simulink model "quadcopter_rotation_subsystem"  (R2023b)
settings: Solver=ode3  StartTime=0  StopTime=inf  FixedStep=0.005  RelTol=1e-3  EnableMultiTasking=on
values from neighbouring files (symbols this model uses):
  alpha_vect = A\B    [poly3traj.m]
  g = 9.81    [MRB.m]
  Ic = [Ixx,0,0;0,Iyy,0;0,0,Izz]    [MRB.m]
  m = 4    [MRB.m]
  Mrb = [m*eye(3),zeros(3);zeros(3),Ic]    [MRB.m]
libraries: aerolibutil x11, simulink_extras x10, slpidlib x6, sharedtransform x3, sharedutil x2, vrlib x2
(part 1 of 2)
settings Model: Creator=The MathWorks, Inc.  LastModifiedBy=branko
settings SolverCC: AlgebraicLoopSolver=TrustRegion
settings DataIOCC: LimitDataPoints=on  SaveFormat=Array  SaveOutput=off  SignalLogging=off  DSMLogging=off  SaveTime=off  ReturnWorkspaceOutputs=off
settings OptimizationCC: BlockReduction=off  BufferReuse=off  LifeSpan=inf
settings DebuggingCC: AlgebraicLoopMsg=none  ParameterPrecisionLossMsg=none  AllowSymbolicDim=off  PregeneratedLibrarySubsystemCodeDiagnostic=none  SFUnexpectedBacktrackingDiag=warning  SFNoUnconditionalDefaultTransitionDiag=warning  SFExecutionAtInitializationDiag=none  ArithmeticOperatorsInVariantConditions=warning
settings HardwareCC: ProdBitPerPointer=32  ProdBitPerSizeT=32  ProdBitPerPtrDiffT=32  ProdLargestAtomicFloat=None  ProdIntDivRoundTo=Undefined  ProdEndianess=Unspecified  ProdWordSize=32  ProdHWDeviceType=32-bit Generic
settings ModelReferenceCC: EnableRefExpFcnMdlSchedulingChecks=on  PropagateSignalLabelsOutOfModel=off
settings SFSimCC: SimUseLocalCustomCode=off  CustomCodeUndefinedFunction=UseInterfaceOnly
settings RTWCC: RTWUseLocalCustomCode=off  DLArmComputeVersion=19.05
settings CodeAppCC: StateflowObjectComments=on
settings GRTTargetCC: TargetLangStandard=C89/C90 (ANSI)
settings ConfigComp: CovMetricSettings=dw  CovSaveCumulativeToWorkspaceVar=on  CovSaveSingleToWorkspaceVar=on  CovExternalEMLEnable=off  CovSFcnEnable=off

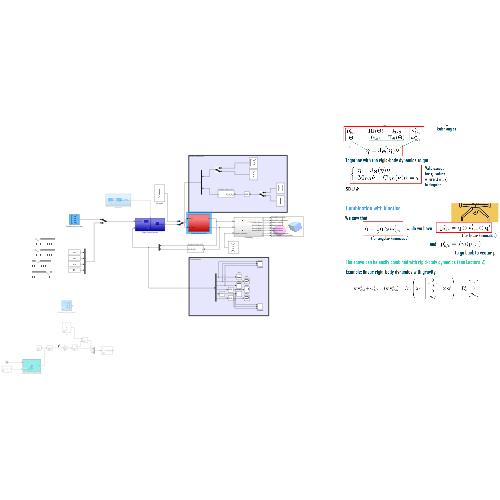
[thumbnail: Simulink's stored preview of the top-level diagram]
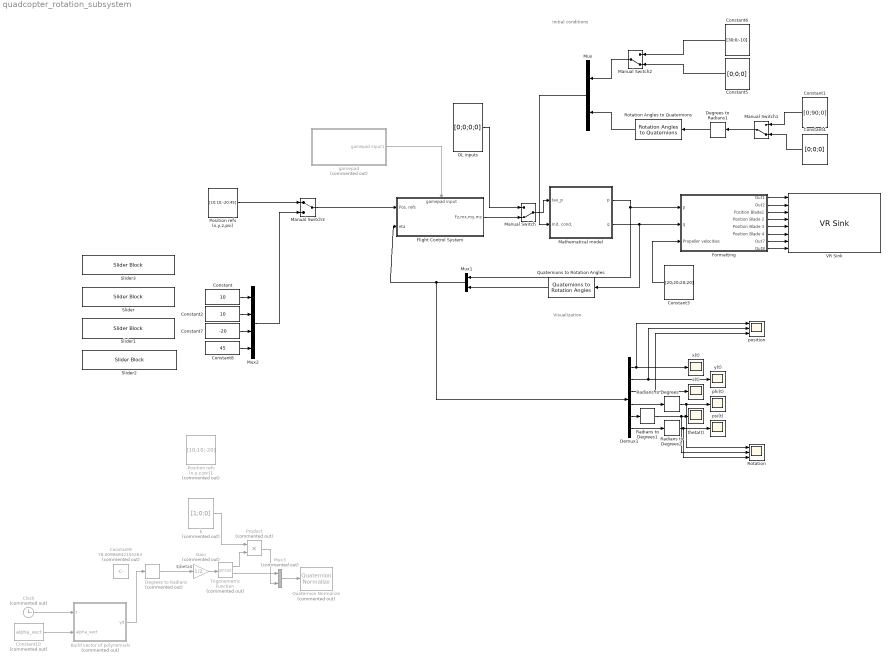
== system quadcopter_rotation_subsystem ==
  note: Visualization
  note: Initial conditions
  note: $\beta$
  Build vector of polynomials : MATLAB Function  Commented=on  TreatAsAtomicUnit=on
  Clock : Clock  Commented=on
  Constant : Constant  Value=10
  Constant1 : Constant  Value=[0;90;0]  VectorParams1D=off
  Constant10 : Constant  Commented=on  Value=alpha_vect  VectorParams1D=off
  Constant2 : Constant  Value=10
  Constant3 : Constant  Value=[20;20;20;20]  VectorParams1D=off
  Constant4 : Constant  Value=[0;0;0]  VectorParams1D=off
  Constant5 : Constant  Value=[0;0;0]  VectorParams1D=off
  Constant6 : Constant  Value=[30;0;-10]  VectorParams1D=off
  Constant7 : Constant  Value=-20
  Constant8 : Constant  Value=45
  Constant9 : Constant  Commented=on  Value=78.00986842105263
  Degrees to Radians : simulink_extras/Transformations/Degrees to Radians  Commented=on
  Degrees to Radians1 : simulink_extras/Transformations/Degrees to Radians
  Demux1 : Demux  Outputs=6
  Flight Control System : Subsystem
      settings: PortSchema="{\"entries\":[{\"content\":{\"sides\":[{\"content\":{\"connectorIds\":[\"In1\",\"In2\"]},\"type\":\"ConnectorPlacement.EquallySpacedRectSide\",\"uuid\":\"8ffec179-99fb-4b4c-a09d-a73fa0154dea\"},{\"content\":{\"connectorIds\":[\"Out1\"],\"side\":\"RIGHT\"},\"type\":\"ConnectorPlacement.EquallySpacedRectSide\",\"uuid\":\"b9ff487d-1da1-449a-81c9-f1838b0d3727\"},{\"content\":{\"connectorIds\":[\"In3\"],\"side\":\"TOP\"},\"type\":\"ConnectorPlacement.EquallySpacedRectSide\",\"uuid\":\"1948ac9a-8b1f-4a62-833b-18e2b106d39d\"}]},\"type\":\"ConnectorPlacement.EquallySpacedConnector\",\"uuid\":\"fea635f7-9753-4696-bad7-e2485c1b5acc\"}],\"packageUris\":[\"http://schema.mathworks.com/mf0/Connector/R2020b\"],\"version\":\"1.0\"}"
  Formatting : Subsystem
  Gain : Gain  Commented=on  Gain=1/2
  Manual Switch : ManualSwitch  CurrentSetting=0
  Manual Switch1 : ManualSwitch  CurrentSetting=0
  Manual Switch2 : ManualSwitch  CurrentSetting=0
  Manual Switch3 : ManualSwitch
  Mathematical model : Subsystem
  Mux : Mux  Inputs=2
  Mux1 : Mux  Inputs=2
  Mux2 : Mux
  Mux3 : Mux  Commented=on  Inputs=2
  OL inputs : Constant  Value=[0;0;0;0]  VectorParams1D=off
  Position refs (x,y,z,psi) : Constant  Value=[10;10;-20;45]  VectorParams1D=off
  Position refs (x,y,z,psi)1 : Constant  Commented=on  Value=[10;10;-20]  VectorParams1D=off
  Product : Product  Commented=on
  Quaternion Normalize : sharedutil/Quaternion Normalize  Commented=on  aMode=aMode
  Quaternions to Rotation Angles : sharedtransform/Quaternions to Rotation Angles  rotationOrder=XYZ  aMode=aMode
  Radians to Degrees : simulink_extras/Transformations/Radians to Degrees
  Radians to Degrees1 : simulink_extras/Transformations/Radians to Degrees
  Radians to Degrees2 : simulink_extras/Transformations/Radians to Degrees
  Rotation : Scope  NumInputPorts=3
  Rotation Angles to Quaternions : sharedtransform/Rotation Angles to Quaternions  rotationOrder=XYZ  aMode=aMode
  Slider : SliderBlock
  Slider1 : SliderBlock  ScaleMin=-50  ScaleMax=50
  Slider2 : SliderBlock  ScaleMin=-65  ScaleMax=65
  Slider3 : SliderBlock
  Trigonometric Function : Trigonometry  Commented=on  Operator=sincos
  VR Sink : vrlib/VR Sink  InstantiateOnLoad=on  SampleTime=12*0.005  ViewEnable=on  RemoteChange=off  RemoteView=off  FieldsWritten=QuadBody.rotation.4.1.1.double#QuadBody.translation.3.1.1.double#Blade1.rotation.4.1.1.double#Blade3.rotation.4.1.1.double#Blade2.rotation.4.1.1.double#Blade4.rotation.4.1.1.double#IsoNoRotation.position.3.1.1.double#OnQuadNoRotation.position.3.1.1.double  WorldFileName=Quadcopter_VR.wrl  AutoView=on  VideoDimensions=[]  AllowVariableSize=off
  gamepad : Subsystem  Commented=on
  k : Constant  Commented=on  Value=[1;0;0]  VectorParams1D=off
  phi(t) : Scope
  position : Scope  NumInputPorts=3
  psi(t) : Scope
  theta(t) : Scope
  x(t) : Scope
  y(t) : Scope
  z(t) : Scope
  wires:
  Formatting/5(Position Blade 3) -> VR Sink/5
  Formatting/7(Out7) -> VR Sink/7
  Formatting/6(Position Blade 4) -> VR Sink/6
  Formatting/3(Position Blade1) -> VR Sink/3
  Formatting/1(Out1) -> VR Sink/1
  Formatting/4(Position Blade 2) -> VR Sink/4
  Formatting/2(Out2) -> VR Sink/2
  Formatting/8(Out8) -> VR Sink/8
  Constant3/1 -> Formatting/3(Propeller velocities)
  OL inputs/1 -> Manual Switch/1
  Flight Control System/1(Fz,mx,my,mz) -> Manual Switch/2
  Manual Switch2/1 -> Mux/1
  Rotation Angles to Quaternions/1 -> Mux/2
  gamepad/1(gamepad input1) -> Flight Control System/3(gamepad input)
  Mathematical model/1(p) -> Mux1/1, Formatting/1(p)
  Mathematical model/2(q) -> Formatting/2(q), Quaternions to Rotation Angles/1
  Mux/1 -> Mathematical model/2(Init. cond.)
  Constant6/1 -> Manual Switch2/1
  Constant5/1 -> Manual Switch2/2
  Manual Switch1/1 -> Degrees to Radians1/1
  Degrees to Radians1/1 -> Rotation Angles to Quaternions/1
  Constant1/1 -> Manual Switch1/1
  Constant4/1 -> Manual Switch1/2
  Quaternions to Rotation Angles/1 -> Mux1/2
  Mux1/1 -> Demux1/1, Flight Control System/2(eta)
  Demux1/5 -> Radians to Degrees1/1
  Demux1/6 -> Radians to Degrees2/1
  Demux1/2 -> position/2, y(t)/1
  Demux1/3 -> z(t)/1, position/3
  Radians to Degrees/1 -> Rotation/1, phi(t)/1
  Demux1/1 -> position/1, x(t)/1
  Radians to Degrees1/1 -> Rotation/2, theta(t)/1
  Radians to Degrees2/1 -> Rotation/3, psi(t)/1
  Demux1/4 -> Radians to Degrees/1
  Constant8/1 -> Mux2/4
  Constant7/1 -> Mux2/3
  Constant/1 -> Mux2/1
  Constant2/1 -> Mux2/2
  Mux2/1 -> Manual Switch3/2
  Manual Switch3/1 -> Flight Control System/1(Pos. refs)
  Trigonometric Function/1 -> Product/2
  Build vector of polynomials/1(yd) -> Degrees to Radians/1
  Mux3/1 -> Quaternion Normalize/1
  Trigonometric Function/2 -> Mux3/1
  Constant10/1 -> Build vector of polynomials/2(alpha_vect)
  Product/1 -> Mux3/2
  Clock/1 -> Build vector of polynomials/1(t)
  Gain/1 -> Trigonometric Function/1
  k/1 -> Product/1
  Degrees to Radians/1 -> Gain/1
  Position refs (x,y,z,psi)/1 -> Manual Switch3/1
  Manual Switch/1 -> Mathematical model/1(tau_p)

== system quadcopter_rotation_subsystem/Flight Control System ==
  Pos. refs : Inport
  eta : Inport  Port=2
  gamepad input : Inport  Port=3
  Inner-loop PID controllers : Subsystem
  Manual Switch : ManualSwitch  CurrentSetting=0
  Outer loop position control : Subsystem
  m_y(t) : Scope
  Fz,mx,my,mz : Outport
  wires:
  Inner-loop PID controllers/1(Fz,mx,my,mz) -> Fz,mx,my,mz/1
  Manual Switch/1 -> Inner-loop PID controllers/1(desired z,phi,theta,psi)
  eta/1 -> Outer loop position control/2(eta), Inner-loop PID controllers/2(eta)
  Pos. refs/1 -> Outer loop position control/1(Pos. refs)
  Outer loop position control/1(desired z,phi,theta,psi) -> Manual Switch/2
  gamepad input/1 -> Manual Switch/1

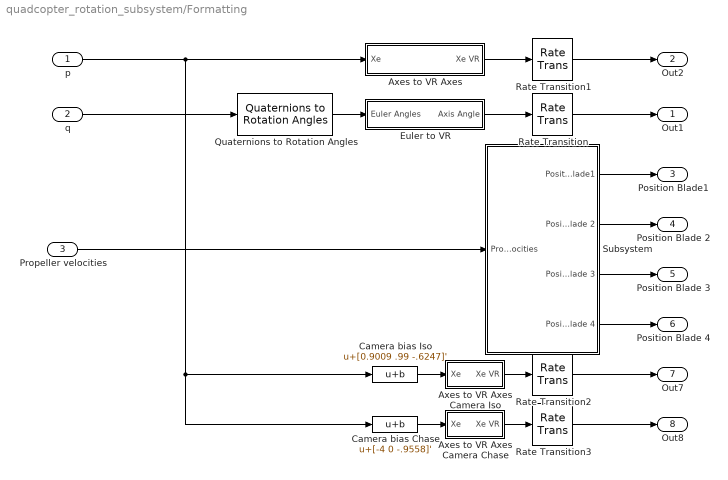
== system quadcopter_rotation_subsystem/Formatting ==
  p : Inport
  q : Inport  Port=2
  Propeller velocities : Inport  Port=3
  Axes to VR Axes : Subsystem
  Axes to VR Axes Camera Chase : Subsystem
  Axes to VR Axes Camera Iso : Subsystem
  Camera bias Chase : Bias  Bias=[-4 0 -.9558]'  SaturateOnIntegerOverflow=off
  Camera bias Iso : Bias  Bias=[0.9009 .99 -.6247]'  SaturateOnIntegerOverflow=off
  Euler to VR : Subsystem
  Quaternions to Rotation Angles : sharedtransform/Quaternions to Rotation Angles  rotationOrder=XYZ  aMode=aMode
  Rate Transition{,1..3} (4 alike) : RateTransition
  Subsystem : Subsystem
  Out1 : Outport
  Out2 : Outport  Port=2
  Position Blade1 : Outport  Port=3
  Position Blade 2 : Outport  Port=4
  Position Blade 3 : Outport  Port=5
  Position Blade 4 : Outport  Port=6
  Out7 : Outport  Port=7
  Out8 : Outport  Port=8
  wires:
  Rate Transition2/1 -> Out7/1
  Propeller velocities/1 -> Subsystem/1(Propeller velocities)
  Subsystem/3(Position Blade 3) -> Position Blade 3/1
  Subsystem/1(Position Blade1) -> Position Blade1/1
  Camera bias Chase/1 -> Axes to VR Axes Camera Chase/1(Xe)
  Axes to VR Axes Camera Chase/1(Xe VR) -> Rate Transition3/1
  Subsystem/2(Position Blade 2) -> Position Blade 2/1
  Axes to VR Axes Camera Iso/1(Xe VR) -> Rate Transition2/1
  Euler to VR/1(Axis Angle) -> Rate Transition/1
  Axes to VR Axes/1(Xe VR) -> Rate Transition1/1
  Rate Transition1/1 -> Out2/1
  Camera bias Iso/1 -> Axes to VR Axes Camera Iso/1(Xe)
  Rate Transition3/1 -> Out8/1
  Rate Transition/1 -> Out1/1
  Subsystem/4(Position Blade 4) -> Position Blade 4/1
  Quaternions to Rotation Angles/1 -> Euler to VR/1(Euler Angles)
  q/1 -> Quaternions to Rotation Angles/1
  p/1 -> Camera bias Chase/1, Camera bias Iso/1, Axes to VR Axes/1(Xe)

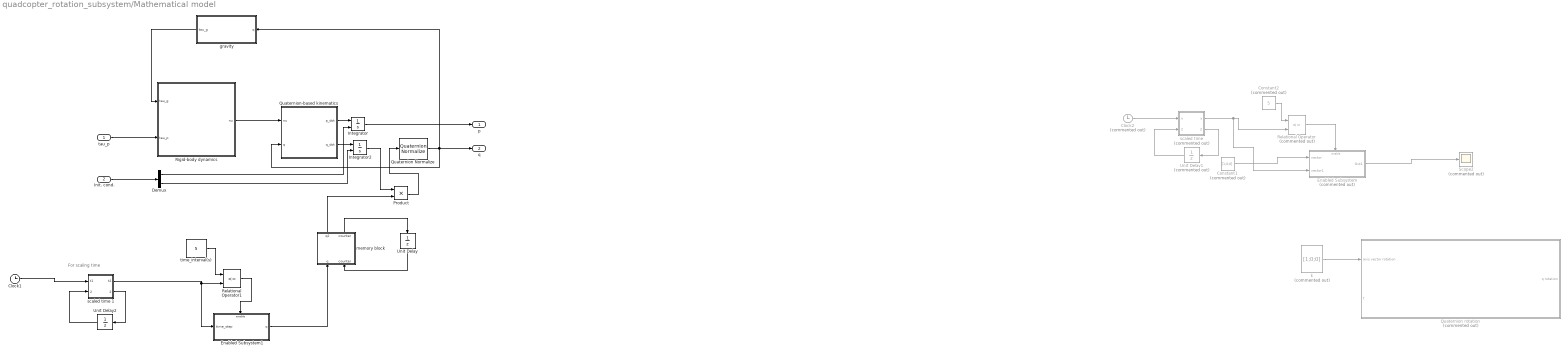
== system quadcopter_rotation_subsystem/Mathematical model ==
  note: For scaling time
  tau_p : Inport
  Init. cond. : Inport  Port=2
  " memory block" : MATLAB Function  TreatAsAtomicUnit=on
  Clock1 : Clock
  Clock2 : Clock  Commented=on
  Constant1 : Constant  Commented=on  Value=[1;0;0]
  Constant2 : Constant  Commented=on  Value=5
  Demux : Demux  Outputs=[3,4]
  Enabled Subsystem : Subsystem  Commented=on  TreatAsAtomicUnit=on
  Enabled Subsystem1 : Subsystem  TreatAsAtomicUnit=on
  Integrator : Integrator  InitialConditionSource=external  InitialCondition=[0;0;-10]
  Integrator2 : Integrator  InitialConditionSource=external  InitialCondition=[0;0;-10;0;pi/2;0]
  Product : Product
  Quaternion Normalize : sharedutil/Quaternion Normalize  aMode=aMode
  "Quaternion rotation " : Subsystem  Commented=on
  Quaternion-based kinematics : Subsystem
  Relational Operator : RelationalOperator  Commented=on  Operator=<=  OutDataTypeStr=boolean  RndMeth=Simplest  InputSameDT=off
  Relational Operator1 : RelationalOperator  Operator=<=  OutDataTypeStr=boolean  RndMeth=Simplest  InputSameDT=off
  Rigid-body dynamics : Subsystem
  Scope2 : Scope  Commented=on
  Unit Delay : UnitDelay  SampleTime=-1  HasFrameUpgradeWarning=on
  Unit Delay1 : UnitDelay  Commented=on  InitialCondition=[0 25]  SampleTime=0.01  HasFrameUpgradeWarning=on
  Unit Delay2 : UnitDelay  InitialCondition=[0 5]  SampleTime=-1  HasFrameUpgradeWarning=on
  gravity : Subsystem
  k : Constant  Commented=on  Value=[1;0;0]  VectorParams1D=off
  "scaled time " : MATLAB Function  Commented=on  TreatAsAtomicUnit=on
  scaled time 1 : MATLAB Function  TreatAsAtomicUnit=on
  time_interval(s) : Constant  Value=5
  p : Outport
  q : Outport  Port=2
  wires:
  Integrator/1 -> p/1
  Quaternion-based kinematics/1(p_dot) -> Integrator/1
  Quaternion Normalize/1 -> gravity/1(q), q/1, Quaternion-based kinematics/2(q)
  tau_p/1 -> Rigid-body dynamics/2(tau_p)
  Rigid-body dynamics/1(nu) -> Quaternion-based kinematics/1(nu)
  gravity/1(tau_g) -> Rigid-body dynamics/1(tau_g)
  Init. cond./1 -> Demux/1
  Demux/2 -> Integrator2/2
  Demux/1 -> Integrator/2
  Quaternion-based kinematics/2(q_dot) -> Integrator2/1
  Constant2/1 -> Relational Operator/1
  Enabled Subsystem/1(Out1) -> Scope2/1
  Unit Delay1/1 -> "scaled time "/2("counter_timer ")
  Relational Operator/1 -> Enabled Subsystem/Enable
  "scaled time "/1(y) -> Enabled Subsystem/2(vector1), Relational Operator/2
  "scaled time "/2(counter_timer) -> Unit Delay1/1
  Constant1/1 -> Enabled Subsystem/1(vector)
  Clock2/1 -> "scaled time "/1(u)
  k/1 -> "Quaternion rotation "/1(axis vector rotation)
  Clock1/1 -> scaled time 1/1(t1)
  time_interval(s)/1 -> Relational Operator1/1
  Relational Operator1/1 -> Enabled Subsystem1/Enable
  scaled time 1/1(t2) -> Enabled Subsystem1/1(time_step), Relational Operator1/2
  scaled time 1/2(counter_timer) -> Unit Delay2/1
  Unit Delay2/1 -> scaled time 1/2("counter_timer ")
  Enabled Subsystem1/1(q) -> " memory block"/1(q)
  Product/1 -> Quaternion Normalize/1
  Integrator2/1 -> Product/1
  " memory block"/1(q2) -> Product/2
  Unit Delay/1 -> " memory block"/2("counter ")
  " memory block"/2(counter) -> Unit Delay/1

== system quadcopter_rotation_subsystem/gamepad ==
  Formatting1 : Subsystem
  Gamepad1 : vrlib/Joystick Input  joyid=1  adjustports=on  forcefeed=off
  gamepad input1 : Outport
  wires:
  ? -> Formatting1/3(Point of View)
  Gamepad1/1 -> Formatting1/1(Axes)
  Formatting1/1(gamepad input) -> gamepad input1/1
  Gamepad1/2 -> Formatting1/2(Buttons)

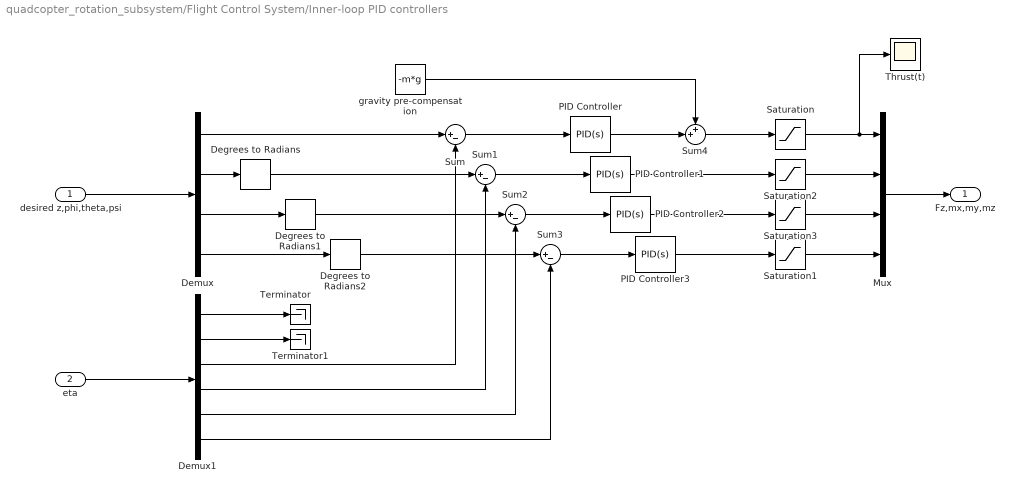
== system quadcopter_rotation_subsystem/Flight Control System/Inner-loop PID controllers ==
  desired z,phi,theta,psi : Inport
  eta : Inport  Port=2
  Degrees to Radians : simulink_extras/Transformations/Degrees to Radians
  Degrees to Radians1 : simulink_extras/Transformations/Degrees to Radians
  Degrees to Radians2 : simulink_extras/Transformations/Degrees to Radians
  Demux : Demux
  Demux1 : Demux  Outputs=6
  Mux : Mux
  PID Controller : slpidlib/PID Controller  Controller=PID  Form=Parallel  TimeDomain=Continuous-time  UseExternalTs=off  SampleTime=-1  IntegratorMethod=Forward Euler  FilterMethod=Forward Euler  ControllerParametersSource=internal  P=0.742717053084559  I=0.0347701341647605  UseKiTs=off  D=3.89568392639278  N=5.45397025421619  UseFilter=on  TunerSelectOption=Transfer Function Based (PID Tuner App)  InitialConditionSource=internal  InitialConditionForIntegrator=0  InitialConditionForFilter=0  DifferentiatorICPrevScaledInput=0  ExternalReset=none  TrackingMode=off  Kt=1  LimitOutput=off  SatLimitsSource=internal  UpperSaturationLimit=100  LowerSaturationLimit=-100  LinearizeAsGain=on  AntiWindupMode=none  Kb=1  LimitIntegrator=off  UpperIntegratorSaturationLimit=inf  LowerIntegratorSaturationLimit=-inf  POutMin=[]  POutMax=[]  IOutMin=[]  IOutMax=[]  DOutMin=[]  DOutMax=[]  NOutMin=[]  NOutMax=[]  SumOutMin=[]  SumOutMax=[]  SaturationOutMin=[]  SaturationOutMax=[]  PParamMin=[]  PParamMax=[]  IParamMin=[]  IParamMax=[]  DParamMin=[]  DParamMax=[]  NParamMin=[]  NParamMax=[]  KbParamMin=[]  KbParamMax=[]  KtParamMin=[]  KtParamMax=[]  KbOutMin=[]  KbOutMax=[]  KtOutMin=[]  KtOutMax=[]  IntegratorOutMin=[]  IntegratorOutMax=[]  FilterOutMin=[]  FilterOutMax=[]  SumI1OutMin=[]  SumI1OutMax=[]  SumI2OutMin=[]  SumI2OutMax=[]  SumI3OutMin=[]  SumI3OutMax=[]  SumI4OutMin=[]  SumI4OutMax=[]  SumDOutMin=[]  SumDOutMax=[]  DifferentiatorOutMin=[]  DifferentiatorOutMax=[]  FilterDiffOutCoefMin=[]  FilterDiffOutCoefMax=[]  ReciprocalOutMin=[]  ReciprocalOutMax=[]  SumDenOutMin=[]  SumDenOutMax=[]  SumNumOutMin=[]  SumNumOutMax=[]  DivideOutMin=[]  DivideOutMax=[]  UdiffTsProdOutMin=[]  UdiffTsProdOutMax=[]  NTsProdOutMin=[]  NTsProdOutMax=[]  UintegralTsProdOutMin=[]  UintegralTsProdOutMax=[]  UngainTsProdOutMin=[]  UngainTsProdOutMax=[]  ClampingZeroOutDataTypeStr=Inherit: Inherit via back propagation  ClampingZeroOutMin=[]  ClampingZeroOutMax=[]  FilterDenConstantOutDataTypeStr=Inherit: Inherit via back propagation  FilterDenConstantOutMin=[]  FilterDenConstantOutMax=[]  PCopyOutDataTypeStr=Inherit: Inherit via back propagation  PCopyOutMin=[]  PCopyOutMax=[]  NCopyOutDataTypeStr=Inherit: Inherit via back propagation  NCopyOutMin=[]  NCopyOutMax=[]  IntegratorContinuousStateAttributes=''  IntegratorStateMustResolveToSignalObject=off  IntegratorRTWStateStorageClass=Auto  FilterContinuousStateAttributes=''  FilterStateMustResolveToSignalObject=off  FilterRTWStateStorageClass=Auto  ParallelPVariant=InternalParameters  IdealPVariant=Disabled  IVariant=InternalParameters  DVariant=InternalParameters  IntegratorVariant=Continuous  SatVariant=Disabled  AWVariant=Passthrough  PCopyVariant=Disabled  TRVariant=Disabled  FdbkBlocksVariant=Forward  IdealPFdbkVariant=Disabled  SatFdbkVariant=Disabled  DerivativeFilterVariant=ContFilter  NVariant=InternalParameters  NCopyVariant=Disabled  FilterICVariant=InternalICsFilter  IntegratorICVariant=InternalICs  ExternalResetVariant=Disabled  TRSumVariant=Passthrough  SumFdbkVariant=Disabled  SumVariant=Sum_PID  TsampFilterVariant=InternalTs  TsampNgainVariant=Passthrough  TsampIntegralVariant=Disabled_SignalSpec  ExternalSaturationOutDataTypeStr=Inherit: Same as second input
  PID Controller1 : slpidlib/PID Controller  Controller=PID  Form=Parallel  TimeDomain=Continuous-time  UseExternalTs=off  SampleTime=-1  IntegratorMethod=Forward Euler  FilterMethod=Forward Euler  ControllerParametersSource=internal  P=38.1552916307711  I=12.5176201301645  UseKiTs=off  D=17.8958394627173  N=96.5468649773944  UseFilter=on  TunerSelectOption=Transfer Function Based (PID Tuner App)  InitialConditionSource=internal  InitialConditionForIntegrator=0  InitialConditionForFilter=0  DifferentiatorICPrevScaledInput=0  ExternalReset=none  TrackingMode=off  Kt=1  LimitOutput=off  SatLimitsSource=internal  UpperSaturationLimit=inf  LowerSaturationLimit=-inf  LinearizeAsGain=on  AntiWindupMode=none  Kb=1  LimitIntegrator=off  UpperIntegratorSaturationLimit=inf  LowerIntegratorSaturationLimit=-inf  POutMin=[]  POutMax=[]  IOutMin=[]  IOutMax=[]  DOutMin=[]  DOutMax=[]  NOutMin=[]  NOutMax=[]  SumOutMin=[]  SumOutMax=[]  SaturationOutMin=[]  SaturationOutMax=[]  PParamMin=[]  PParamMax=[]  IParamMin=[]  IParamMax=[]  DParamMin=[]  DParamMax=[]  NParamMin=[]  NParamMax=[]  KbParamMin=[]  KbParamMax=[]  KtParamMin=[]  KtParamMax=[]  KbOutMin=[]  KbOutMax=[]  KtOutMin=[]  KtOutMax=[]  IntegratorOutMin=[]  IntegratorOutMax=[]  FilterOutMin=[]  FilterOutMax=[]  SumI1OutMin=[]  SumI1OutMax=[]  SumI2OutMin=[]  SumI2OutMax=[]  SumI3OutMin=[]  SumI3OutMax=[]  SumI4OutMin=[]  SumI4OutMax=[]  SumDOutMin=[]  SumDOutMax=[]  DifferentiatorOutMin=[]  DifferentiatorOutMax=[]  FilterDiffOutCoefMin=[]  FilterDiffOutCoefMax=[]  ReciprocalOutMin=[]  ReciprocalOutMax=[]  SumDenOutMin=[]  SumDenOutMax=[]  SumNumOutMin=[]  SumNumOutMax=[]  DivideOutMin=[]  DivideOutMax=[]  UdiffTsProdOutMin=[]  UdiffTsProdOutMax=[]  NTsProdOutMin=[]  NTsProdOutMax=[]  UintegralTsProdOutMin=[]  UintegralTsProdOutMax=[]  UngainTsProdOutMin=[]  UngainTsProdOutMax=[]  ClampingZeroOutDataTypeStr=Inherit: Inherit via back propagation  ClampingZeroOutMin=[]  ClampingZeroOutMax=[]  FilterDenConstantOutDataTypeStr=Inherit: Inherit via back propagation  FilterDenConstantOutMin=[]  FilterDenConstantOutMax=[]  PCopyOutDataTypeStr=Inherit: Inherit via back propagation  PCopyOutMin=[]  PCopyOutMax=[]  NCopyOutDataTypeStr=Inherit: Inherit via back propagation  NCopyOutMin=[]  NCopyOutMax=[]  IntegratorContinuousStateAttributes=''  IntegratorStateMustResolveToSignalObject=off  IntegratorRTWStateStorageClass=Auto  FilterContinuousStateAttributes=''  FilterStateMustResolveToSignalObject=off  FilterRTWStateStorageClass=Auto  ParallelPVariant=InternalParameters  IdealPVariant=Disabled  IVariant=InternalParameters  DVariant=InternalParameters  IntegratorVariant=Continuous  SatVariant=Disabled  AWVariant=Passthrough  PCopyVariant=Disabled  TRVariant=Disabled  FdbkBlocksVariant=Forward  IdealPFdbkVariant=Disabled  SatFdbkVariant=Disabled  DerivativeFilterVariant=ContFilter  NVariant=InternalParameters  NCopyVariant=Disabled  FilterICVariant=InternalICsFilter  IntegratorICVariant=InternalICs  ExternalResetVariant=Disabled  TRSumVariant=Passthrough  SumFdbkVariant=Disabled  SumVariant=Sum_PID  TsampFilterVariant=InternalTs  TsampNgainVariant=Passthrough  TsampIntegralVariant=Disabled_SignalSpec  ExternalSaturationOutDataTypeStr=Inherit: Same as second input
  PID Controller2 : slpidlib/PID Controller  Controller=PID  Form=Parallel  TimeDomain=Continuous-time  UseExternalTs=off  SampleTime=-1  IntegratorMethod=Forward Euler  FilterMethod=Forward Euler  ControllerParametersSource=internal  P=34.9127173436624  I=10.8701783766729  UseKiTs=off  D=17.1374646672708  N=92.4492805196359  UseFilter=on  TunerSelectOption=Transfer Function Based (PID Tuner App)  InitialConditionSource=internal  InitialConditionForIntegrator=0  InitialConditionForFilter=0  DifferentiatorICPrevScaledInput=0  ExternalReset=none  TrackingMode=off  Kt=1  LimitOutput=off  SatLimitsSource=internal  UpperSaturationLimit=inf  LowerSaturationLimit=-inf  LinearizeAsGain=on  AntiWindupMode=none  Kb=1  LimitIntegrator=off  UpperIntegratorSaturationLimit=inf  LowerIntegratorSaturationLimit=-inf  POutMin=[]  POutMax=[]  IOutMin=[]  IOutMax=[]  DOutMin=[]  DOutMax=[]  NOutMin=[]  NOutMax=[]  SumOutMin=[]  SumOutMax=[]  SaturationOutMin=[]  SaturationOutMax=[]  PParamMin=[]  PParamMax=[]  IParamMin=[]  IParamMax=[]  DParamMin=[]  DParamMax=[]  NParamMin=[]  NParamMax=[]  KbParamMin=[]  KbParamMax=[]  KtParamMin=[]  KtParamMax=[]  KbOutMin=[]  KbOutMax=[]  KtOutMin=[]  KtOutMax=[]  IntegratorOutMin=[]  IntegratorOutMax=[]  FilterOutMin=[]  FilterOutMax=[]  SumI1OutMin=[]  SumI1OutMax=[]  SumI2OutMin=[]  SumI2OutMax=[]  SumI3OutMin=[]  SumI3OutMax=[]  SumI4OutMin=[]  SumI4OutMax=[]  SumDOutMin=[]  SumDOutMax=[]  DifferentiatorOutMin=[]  DifferentiatorOutMax=[]  FilterDiffOutCoefMin=[]  FilterDiffOutCoefMax=[]  ReciprocalOutMin=[]  ReciprocalOutMax=[]  SumDenOutMin=[]  SumDenOutMax=[]  SumNumOutMin=[]  SumNumOutMax=[]  DivideOutMin=[]  DivideOutMax=[]  UdiffTsProdOutMin=[]  UdiffTsProdOutMax=[]  NTsProdOutMin=[]  NTsProdOutMax=[]  UintegralTsProdOutMin=[]  UintegralTsProdOutMax=[]  UngainTsProdOutMin=[]  UngainTsProdOutMax=[]  ClampingZeroOutDataTypeStr=Inherit: Inherit via back propagation  ClampingZeroOutMin=[]  ClampingZeroOutMax=[]  FilterDenConstantOutDataTypeStr=Inherit: Inherit via back propagation  FilterDenConstantOutMin=[]  FilterDenConstantOutMax=[]  PCopyOutDataTypeStr=Inherit: Inherit via back propagation  PCopyOutMin=[]  PCopyOutMax=[]  NCopyOutDataTypeStr=Inherit: Inherit via back propagation  NCopyOutMin=[]  NCopyOutMax=[]  IntegratorContinuousStateAttributes=''  IntegratorStateMustResolveToSignalObject=off  IntegratorRTWStateStorageClass=Auto  FilterContinuousStateAttributes=''  FilterStateMustResolveToSignalObject=off  FilterRTWStateStorageClass=Auto  ParallelPVariant=InternalParameters  IdealPVariant=Disabled  IVariant=InternalParameters  DVariant=InternalParameters  IntegratorVariant=Continuous  SatVariant=Disabled  AWVariant=Passthrough  PCopyVariant=Disabled  TRVariant=Disabled  FdbkBlocksVariant=Forward  IdealPFdbkVariant=Disabled  SatFdbkVariant=Disabled  DerivativeFilterVariant=ContFilter  NVariant=InternalParameters  NCopyVariant=Disabled  FilterICVariant=InternalICsFilter  IntegratorICVariant=InternalICs  ExternalResetVariant=Disabled  TRSumVariant=Passthrough  SumFdbkVariant=Disabled  SumVariant=Sum_PID  TsampFilterVariant=InternalTs  TsampNgainVariant=Passthrough  TsampIntegralVariant=Disabled_SignalSpec  ExternalSaturationOutDataTypeStr=Inherit: Same as second input
  PID Controller3 : slpidlib/PID Controller  Controller=PID  Form=Parallel  TimeDomain=Continuous-time  UseExternalTs=off  SampleTime=-1  IntegratorMethod=Forward Euler  FilterMethod=Forward Euler  ControllerParametersSource=internal  P=0.742717053109316  I=0.0347701341659195  UseKiTs=off  D=3.89568392652263  N=5.45397025421619  UseFilter=on  TunerSelectOption=Transfer Function Based (PID Tuner App)  InitialConditionSource=internal  InitialConditionForIntegrator=0  InitialConditionForFilter=0  DifferentiatorICPrevScaledInput=0  ExternalReset=none  TrackingMode=off  Kt=1  LimitOutput=off  SatLimitsSource=internal  UpperSaturationLimit=inf  LowerSaturationLimit=-inf  LinearizeAsGain=on  AntiWindupMode=none  Kb=1  LimitIntegrator=off  UpperIntegratorSaturationLimit=inf  LowerIntegratorSaturationLimit=-inf  POutMin=[]  POutMax=[]  IOutMin=[]  IOutMax=[]  DOutMin=[]  DOutMax=[]  NOutMin=[]  NOutMax=[]  SumOutMin=[]  SumOutMax=[]  SaturationOutMin=[]  SaturationOutMax=[]  PParamMin=[]  PParamMax=[]  IParamMin=[]  IParamMax=[]  DParamMin=[]  DParamMax=[]  NParamMin=[]  NParamMax=[]  KbParamMin=[]  KbParamMax=[]  KtParamMin=[]  KtParamMax=[]  KbOutMin=[]  KbOutMax=[]  KtOutMin=[]  KtOutMax=[]  IntegratorOutMin=[]  IntegratorOutMax=[]  FilterOutMin=[]  FilterOutMax=[]  SumI1OutMin=[]  SumI1OutMax=[]  SumI2OutMin=[]  SumI2OutMax=[]  SumI3OutMin=[]  SumI3OutMax=[]  SumI4OutMin=[]  SumI4OutMax=[]  SumDOutMin=[]  SumDOutMax=[]  DifferentiatorOutMin=[]  DifferentiatorOutMax=[]  FilterDiffOutCoefMin=[]  FilterDiffOutCoefMax=[]  ReciprocalOutMin=[]  ReciprocalOutMax=[]  SumDenOutMin=[]  SumDenOutMax=[]  SumNumOutMin=[]  SumNumOutMax=[]  DivideOutMin=[]  DivideOutMax=[]  UdiffTsProdOutMin=[]  UdiffTsProdOutMax=[]  NTsProdOutMin=[]  NTsProdOutMax=[]  UintegralTsProdOutMin=[]  UintegralTsProdOutMax=[]  UngainTsProdOutMin=[]  UngainTsProdOutMax=[]  ClampingZeroOutDataTypeStr=Inherit: Inherit via back propagation  ClampingZeroOutMin=[]  ClampingZeroOutMax=[]  FilterDenConstantOutDataTypeStr=Inherit: Inherit via back propagation  FilterDenConstantOutMin=[]  FilterDenConstantOutMax=[]  PCopyOutDataTypeStr=Inherit: Inherit via back propagation  PCopyOutMin=[]  PCopyOutMax=[]  NCopyOutDataTypeStr=Inherit: Inherit via back propagation  NCopyOutMin=[]  NCopyOutMax=[]  IntegratorContinuousStateAttributes=''  IntegratorStateMustResolveToSignalObject=off  IntegratorRTWStateStorageClass=Auto  FilterContinuousStateAttributes=''  FilterStateMustResolveToSignalObject=off  FilterRTWStateStorageClass=Auto  ParallelPVariant=InternalParameters  IdealPVariant=Disabled  IVariant=InternalParameters  DVariant=InternalParameters  IntegratorVariant=Continuous  SatVariant=Disabled  AWVariant=Passthrough  PCopyVariant=Disabled  TRVariant=Disabled  FdbkBlocksVariant=Forward  IdealPFdbkVariant=Disabled  SatFdbkVariant=Disabled  DerivativeFilterVariant=ContFilter  NVariant=InternalParameters  NCopyVariant=Disabled  FilterICVariant=InternalICsFilter  IntegratorICVariant=InternalICs  ExternalResetVariant=Disabled  TRSumVariant=Passthrough  SumFdbkVariant=Disabled  SumVariant=Sum_PID  TsampFilterVariant=InternalTs  TsampNgainVariant=Passthrough  TsampIntegralVariant=Disabled_SignalSpec  ExternalSaturationOutDataTypeStr=Inherit: Same as second input
  Saturation{,1..3} (4 alike) : Saturate  UpperLimit=100  LowerLimit=-100
  Sum{,1..3} (4 alike) : Sum  Inputs=|+-
  Sum4 : Sum  Inputs=++|
  Terminator : Terminator
  Terminator1 : Terminator
  Thrust(t) : Scope
  gravity pre-compensation : Constant  Value=-m*g
  Fz,mx,my,mz : Outport
  wires:
  Mux/1 -> Fz,mx,my,mz/1
  Sum/1 -> PID Controller/1
  Sum1/1 -> PID Controller1/1
  PID Controller1/1 -> Saturation2/1
  PID Controller2/1 -> Saturation3/1
  PID Controller3/1 -> Saturation1/1
  Sum2/1 -> PID Controller2/1
  Sum3/1 -> PID Controller3/1
  Demux/2 -> Degrees to Radians/1
  Demux/3 -> Degrees to Radians1/1
  Demux/4 -> Degrees to Radians2/1
  desired z,phi,theta,psi/1 -> Demux/1
  eta/1 -> Demux1/1
  Demux1/1 -> Terminator/1
  Demux1/2 -> Terminator1/1
  Demux1/3 -> Sum/2
  Demux1/4 -> Sum1/2
  Demux1/5 -> Sum2/2
  Demux1/6 -> Sum3/2
  Degrees to Radians/1 -> Sum1/1
  Degrees to Radians1/1 -> Sum2/1
  Degrees to Radians2/1 -> Sum3/1
  Demux/1 -> Sum/1
  Saturation/1 -> Thrust(t)/1, Mux/1
  Saturation1/1 -> Mux/4
  Saturation2/1 -> Mux/2
  Saturation3/1 -> Mux/3
  gravity pre-compensation/1 -> Sum4/1
  Sum4/1 -> Saturation/1
  PID Controller/1 -> Sum4/2

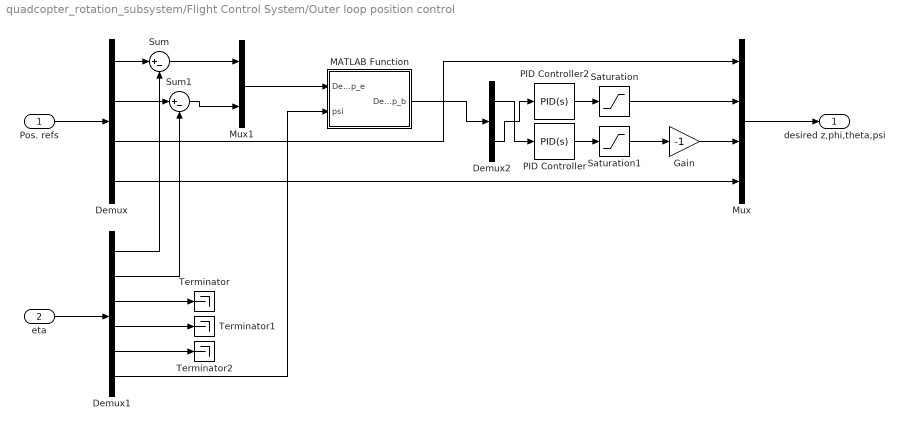
== system quadcopter_rotation_subsystem/Flight Control System/Outer loop position control ==
  Pos. refs : Inport
  eta : Inport  Port=2
  Demux : Demux
  Demux1 : Demux  Outputs=6
  Demux2 : Demux  Outputs=2
  Gain : Gain  Gain=-1
  MATLAB Function : MATLAB Function  TreatAsAtomicUnit=on
  Mux : Mux
  Mux1 : Mux  Inputs=2
  PID Controller : slpidlib/PID Controller  Controller=PID  Form=Parallel  TimeDomain=Continuous-time  UseExternalTs=off  SampleTime=-1  IntegratorMethod=Forward Euler  FilterMethod=Forward Euler  ControllerParametersSource=internal  P=-0.0479842809986179  I=-0.000156936561948268  UseKiTs=off  D=-2.47277772854368  N=54.3882327003062  UseFilter=on  TunerSelectOption=Transfer Function Based (PID Tuner App)  InitialConditionSource=internal  InitialConditionForIntegrator=0  InitialConditionForFilter=0  DifferentiatorICPrevScaledInput=0  ExternalReset=none  TrackingMode=off  Kt=1  LimitOutput=off  SatLimitsSource=internal  UpperSaturationLimit=100  LowerSaturationLimit=-100  LinearizeAsGain=on  AntiWindupMode=none  Kb=1  LimitIntegrator=off  UpperIntegratorSaturationLimit=inf  LowerIntegratorSaturationLimit=-inf  POutMin=[]  POutMax=[]  IOutMin=[]  IOutMax=[]  DOutMin=[]  DOutMax=[]  NOutMin=[]  NOutMax=[]  SumOutMin=[]  SumOutMax=[]  SaturationOutMin=[]  SaturationOutMax=[]  PParamMin=[]  PParamMax=[]  IParamMin=[]  IParamMax=[]  DParamMin=[]  DParamMax=[]  NParamMin=[]  NParamMax=[]  KbParamMin=[]  KbParamMax=[]  KtParamMin=[]  KtParamMax=[]  KbOutMin=[]  KbOutMax=[]  KtOutMin=[]  KtOutMax=[]  IntegratorOutMin=[]  IntegratorOutMax=[]  FilterOutMin=[]  FilterOutMax=[]  SumI1OutMin=[]  SumI1OutMax=[]  SumI2OutMin=[]  SumI2OutMax=[]  SumI3OutMin=[]  SumI3OutMax=[]  SumI4OutMin=[]  SumI4OutMax=[]  SumDOutMin=[]  SumDOutMax=[]  DifferentiatorOutMin=[]  DifferentiatorOutMax=[]  FilterDiffOutCoefMin=[]  FilterDiffOutCoefMax=[]  ReciprocalOutMin=[]  ReciprocalOutMax=[]  SumDenOutMin=[]  SumDenOutMax=[]  SumNumOutMin=[]  SumNumOutMax=[]  DivideOutMin=[]  DivideOutMax=[]  UdiffTsProdOutMin=[]  UdiffTsProdOutMax=[]  NTsProdOutMin=[]  NTsProdOutMax=[]  UintegralTsProdOutMin=[]  UintegralTsProdOutMax=[]  UngainTsProdOutMin=[]  UngainTsProdOutMax=[]  ClampingZeroOutDataTypeStr=Inherit: Inherit via back propagation  ClampingZeroOutMin=[]  ClampingZeroOutMax=[]  FilterDenConstantOutDataTypeStr=Inherit: Inherit via back propagation  FilterDenConstantOutMin=[]  FilterDenConstantOutMax=[]  PCopyOutDataTypeStr=Inherit: Inherit via back propagation  PCopyOutMin=[]  PCopyOutMax=[]  NCopyOutDataTypeStr=Inherit: Inherit via back propagation  NCopyOutMin=[]  NCopyOutMax=[]  IntegratorContinuousStateAttributes=''  IntegratorStateMustResolveToSignalObject=off  IntegratorRTWStateStorageClass=Auto  FilterContinuousStateAttributes=''  FilterStateMustResolveToSignalObject=off  FilterRTWStateStorageClass=Auto  ParallelPVariant=InternalParameters  IdealPVariant=Disabled  IVariant=InternalParameters  DVariant=InternalParameters  IntegratorVariant=Continuous  SatVariant=Disabled  AWVariant=Passthrough  PCopyVariant=Disabled  TRVariant=Disabled  FdbkBlocksVariant=Forward  IdealPFdbkVariant=Disabled  SatFdbkVariant=Disabled  DerivativeFilterVariant=ContFilter  NVariant=InternalParameters  NCopyVariant=Disabled  FilterICVariant=InternalICsFilter  IntegratorICVariant=InternalICs  ExternalResetVariant=Disabled  TRSumVariant=Passthrough  SumFdbkVariant=Disabled  SumVariant=Sum_PID  TsampFilterVariant=InternalTs  TsampNgainVariant=Passthrough  TsampIntegralVariant=Disabled_SignalSpec  ExternalSaturationOutDataTypeStr=Inherit: Same as second input
  PID Controller2 : slpidlib/PID Controller  Controller=PID  Form=Parallel  TimeDomain=Continuous-time  UseExternalTs=off  SampleTime=-1  IntegratorMethod=Forward Euler  FilterMethod=Forward Euler  ControllerParametersSource=internal  P=-0.0341447952127922  I=-9.92681041052417e-05  UseKiTs=off  D=-2.60951782930978  N=56.9514711385266  UseFilter=on  TunerSelectOption=Transfer Function Based (PID Tuner App)  InitialConditionSource=internal  InitialConditionForIntegrator=0  InitialConditionForFilter=0  DifferentiatorICPrevScaledInput=0  ExternalReset=none  TrackingMode=off  Kt=1  LimitOutput=off  SatLimitsSource=internal  UpperSaturationLimit=100  LowerSaturationLimit=-100  LinearizeAsGain=on  AntiWindupMode=none  Kb=1  LimitIntegrator=off  UpperIntegratorSaturationLimit=inf  LowerIntegratorSaturationLimit=-inf  POutMin=[]  POutMax=[]  IOutMin=[]  IOutMax=[]  DOutMin=[]  DOutMax=[]  NOutMin=[]  NOutMax=[]  SumOutMin=[]  SumOutMax=[]  SaturationOutMin=[]  SaturationOutMax=[]  PParamMin=[]  PParamMax=[]  IParamMin=[]  IParamMax=[]  DParamMin=[]  DParamMax=[]  NParamMin=[]  NParamMax=[]  KbParamMin=[]  KbParamMax=[]  KtParamMin=[]  KtParamMax=[]  KbOutMin=[]  KbOutMax=[]  KtOutMin=[]  KtOutMax=[]  IntegratorOutMin=[]  IntegratorOutMax=[]  FilterOutMin=[]  FilterOutMax=[]  SumI1OutMin=[]  SumI1OutMax=[]  SumI2OutMin=[]  SumI2OutMax=[]  SumI3OutMin=[]  SumI3OutMax=[]  SumI4OutMin=[]  SumI4OutMax=[]  SumDOutMin=[]  SumDOutMax=[]  DifferentiatorOutMin=[]  DifferentiatorOutMax=[]  FilterDiffOutCoefMin=[]  FilterDiffOutCoefMax=[]  ReciprocalOutMin=[]  ReciprocalOutMax=[]  SumDenOutMin=[]  SumDenOutMax=[]  SumNumOutMin=[]  SumNumOutMax=[]  DivideOutMin=[]  DivideOutMax=[]  UdiffTsProdOutMin=[]  UdiffTsProdOutMax=[]  NTsProdOutMin=[]  NTsProdOutMax=[]  UintegralTsProdOutMin=[]  UintegralTsProdOutMax=[]  UngainTsProdOutMin=[]  UngainTsProdOutMax=[]  ClampingZeroOutDataTypeStr=Inherit: Inherit via back propagation  ClampingZeroOutMin=[]  ClampingZeroOutMax=[]  FilterDenConstantOutDataTypeStr=Inherit: Inherit via back propagation  FilterDenConstantOutMin=[]  FilterDenConstantOutMax=[]  PCopyOutDataTypeStr=Inherit: Inherit via back propagation  PCopyOutMin=[]  PCopyOutMax=[]  NCopyOutDataTypeStr=Inherit: Inherit via back propagation  NCopyOutMin=[]  NCopyOutMax=[]  IntegratorContinuousStateAttributes=''  IntegratorStateMustResolveToSignalObject=off  IntegratorRTWStateStorageClass=Auto  FilterContinuousStateAttributes=''  FilterStateMustResolveToSignalObject=off  FilterRTWStateStorageClass=Auto  ParallelPVariant=InternalParameters  IdealPVariant=Disabled  IVariant=InternalParameters  DVariant=InternalParameters  IntegratorVariant=Continuous  SatVariant=Disabled  AWVariant=Passthrough  PCopyVariant=Disabled  TRVariant=Disabled  FdbkBlocksVariant=Forward  IdealPFdbkVariant=Disabled  SatFdbkVariant=Disabled  DerivativeFilterVariant=ContFilter  NVariant=InternalParameters  NCopyVariant=Disabled  FilterICVariant=InternalICsFilter  IntegratorICVariant=InternalICs  ExternalResetVariant=Disabled  TRSumVariant=Passthrough  SumFdbkVariant=Disabled  SumVariant=Sum_PID  TsampFilterVariant=InternalTs  TsampNgainVariant=Passthrough  TsampIntegralVariant=Disabled_SignalSpec  ExternalSaturationOutDataTypeStr=Inherit: Same as second input
  Saturation : Saturate  UpperLimit=5  LowerLimit=-5
  Saturation1 : Saturate  UpperLimit=5  LowerLimit=-5
  Sum : Sum  Inputs=|+-
  Sum1 : Sum  Inputs=|+-
  Terminator : Terminator
  Terminator1 : Terminator
  Terminator2 : Terminator
  desired z,phi,theta,psi : Outport
  wires:
  Demux1/3 -> Terminator/1
  Demux1/5 -> Terminator2/1
  Pos. refs/1 -> Demux/1
  Demux1/2 -> Sum1/2
  Demux1/4 -> Terminator1/1
  Demux1/1 -> Sum/2
  eta/1 -> Demux1/1
  Mux/1 -> desired z,phi,theta,psi/1
  PID Controller/1 -> Saturation1/1
  PID Controller2/1 -> Saturation/1
  Saturation1/1 -> Gain/1
  Gain/1 -> Mux/3
  Saturation/1 -> Mux/2
  Demux/3 -> Mux/1
  Demux/4 -> Mux/4
  Demux/1 -> Sum/1
  Demux/2 -> Sum1/1
  Sum/1 -> Mux1/1
  Sum1/1 -> Mux1/2
  MATLAB Function/1(Deltap_b) -> Demux2/1
  Mux1/1 -> MATLAB Function/1(Deltap_e)
  Demux1/6 -> MATLAB Function/2(psi)
  Demux2/1 -> PID Controller/1
  Demux2/2 -> PID Controller2/1

== system quadcopter_rotation_subsystem/Formatting/Axes to VR Axes ==
  Xe : Inport
  Demux : Demux  Outputs=3
      settings: DisplayOption=none
  Mux : Mux  Inputs=3
  rad-->deg1 : Gain  Gain=-1  SaturateOnIntegerOverflow=on  OutDataTypeStr=Inherit: Same as input  ParamDataTypeStr=Inherit: Same as input
  Xe VR : Outport  VectorParamsAs1DForOutWhenUnconnected=off
  wires:
  Xe/1 -> Demux/1
  Demux/1 -> Mux/1
  Demux/3 -> rad-->deg1/1
  Mux/1 -> Xe VR/1
  rad-->deg1/1 -> Mux/2
  Demux/2 -> Mux/3

== system quadcopter_rotation_subsystem/Formatting/Axes to VR Axes Camera Chase ==
  Xe : Inport
  Demux : Demux  Outputs=3
      settings: DisplayOption=none
  Mux : Mux  Inputs=3
  rad-->deg1 : Gain  Gain=-1  SaturateOnIntegerOverflow=on  OutDataTypeStr=Inherit: Same as input  ParamDataTypeStr=Inherit: Same as input
  Xe VR : Outport  VectorParamsAs1DForOutWhenUnconnected=off
  wires:
  Xe/1 -> Demux/1
  Demux/1 -> Mux/1
  Demux/3 -> rad-->deg1/1
  Mux/1 -> Xe VR/1
  rad-->deg1/1 -> Mux/2
  Demux/2 -> Mux/3

== system quadcopter_rotation_subsystem/Formatting/Axes to VR Axes Camera Iso ==
  Xe : Inport
  Demux : Demux  Outputs=3
      settings: DisplayOption=none
  Mux : Mux  Inputs=3
  rad-->deg1 : Gain  Gain=-1  SaturateOnIntegerOverflow=on  OutDataTypeStr=Inherit: Same as input  ParamDataTypeStr=Inherit: Same as input
  Xe VR : Outport  VectorParamsAs1DForOutWhenUnconnected=off
  wires:
  Demux/2 -> Mux/3
  rad-->deg1/1 -> Mux/2
  Mux/1 -> Xe VR/1
  Demux/3 -> rad-->deg1/1
  Demux/1 -> Mux/1
  Xe/1 -> Demux/1

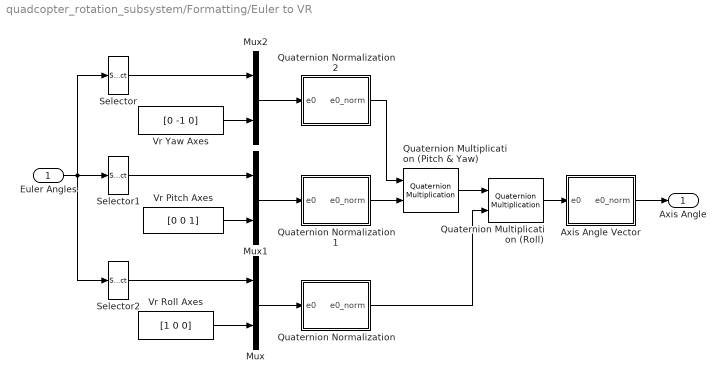
== system quadcopter_rotation_subsystem/Formatting/Euler to VR ==
  Euler Angles : Inport
  Axis Angle Vector : Subsystem
  Mux : Mux  Inputs=2
  Mux1 : Mux  Inputs=2
  Mux2 : Mux  Inputs=2
  Quaternion Multiplication (Pitch & Yaw) : aerolibutil/Quaternion Multiplication
  Quaternion Multiplication (Roll) : aerolibutil/Quaternion Multiplication
  Quaternion Normalization : Subsystem
  Quaternion Normalization1 : Subsystem
  Quaternion Normalization2 : Subsystem
  Selector : Selector  InputPortWidth=3  IndexOptions=Index vector (dialog)  Indices=[3]  OutputSizes=1
  Selector1 : Selector  InputPortWidth=3  IndexOptions=Index vector (dialog)  Indices=[2]  OutputSizes=1
  Selector2 : Selector  InputPortWidth=3  IndexOptions=Index vector (dialog)  Indices=[1]  OutputSizes=1
  Vr Pitch Axes : Constant  Value=[0 0 1]
  Vr Roll Axes : Constant  Value=[1 0 0]
  Vr Yaw Axes : Constant  Value=[0 -1 0]
  Axis Angle : Outport  VectorParamsAs1DForOutWhenUnconnected=off
  wires:
  Quaternion Multiplication (Roll)/1 -> Axis Angle Vector/1(e0)
  Axis Angle Vector/1(e0_norm) -> Axis Angle/1
  Quaternion Normalization/1(e0_norm) -> Quaternion Multiplication (Roll)/2
  Quaternion Normalization2/1(e0_norm) -> Quaternion Multiplication (Pitch & Yaw)/1
  Quaternion Normalization1/1(e0_norm) -> Quaternion Multiplication (Pitch & Yaw)/2
  Mux2/1 -> Quaternion Normalization2/1(e0)
  Mux1/1 -> Quaternion Normalization1/1(e0)
  Mux/1 -> Quaternion Normalization/1(e0)
  Selector/1 -> Mux2/1
  Vr Yaw Axes/1 -> Mux2/2
  Selector1/1 -> Mux1/1
  Vr Pitch Axes/1 -> Mux1/2
  Selector2/1 -> Mux/1
  Vr Roll Axes/1 -> Mux/2
  Euler Angles/1 -> Selector2/1, Selector1/1, Selector/1
  Quaternion Multiplication (Pitch & Yaw)/1 -> Quaternion Multiplication (Roll)/1

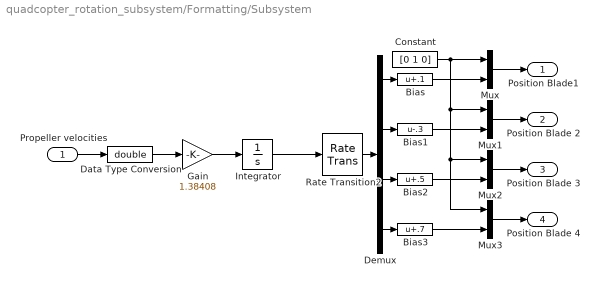
== system quadcopter_rotation_subsystem/Formatting/Subsystem ==
  Propeller velocities : Inport
  Bias : Bias  Bias=.1  SaturateOnIntegerOverflow=off
  Bias1 : Bias  Bias=-.3  SaturateOnIntegerOverflow=off
  Bias2 : Bias  Bias=.5  SaturateOnIntegerOverflow=off
  Bias3 : Bias  Bias=.7  SaturateOnIntegerOverflow=off
  Constant : Constant  Value=[0 1 0]
  Data Type Conversion : DataTypeConversion  OutDataTypeStr=double  SaturateOnIntegerOverflow=off  RndMeth=Floor
  Demux : Demux
  Gain : Gain  Gain=1.38408
  Integrator : Integrator  InitialCondition=[.1 ; .2 ;-.3 ;-.4]  WrapState=on  WrappedStateUpperValue=2*pi  WrappedStateLowerValue=-2*pi
  Mux{,1..3} (4 alike) : Mux  Inputs=2
  Rate Transition2 : RateTransition
  Position Blade1 : Outport  VectorParamsAs1DForOutWhenUnconnected=off
  Position Blade 2 : Outport  Port=2  VectorParamsAs1DForOutWhenUnconnected=off
  Position Blade 3 : Outport  Port=3  VectorParamsAs1DForOutWhenUnconnected=off
  Position Blade 4 : Outport  Port=4  VectorParamsAs1DForOutWhenUnconnected=off
  wires:
  Bias3/1 -> Mux3/2
  Mux3/1 -> Position Blade 4/1
  Bias1/1 -> Mux1/2
  Bias2/1 -> Mux2/2
  Demux/2 -> Bias1/1
  Constant/1 -> Mux3/1, Mux2/1, Mux1/1, Mux/1
  Mux1/1 -> Position Blade 2/1
  Mux2/1 -> Position Blade 3/1
  Integrator/1 -> Rate Transition2/1
  Mux/1 -> Position Blade1/1
  Demux/3 -> Bias2/1
  Bias/1 -> Mux/2
  Propeller velocities/1 -> Data Type Conversion/1
  Demux/4 -> Bias3/1
  Rate Transition2/1 -> Demux/1
  Demux/1 -> Bias/1
  Data Type Conversion/1 -> Gain/1
  Gain/1 -> Integrator/1

== system quadcopter_rotation_subsystem/Mathematical model/Enabled Subsystem ==
  vector : Inport
  vector1 : Inport  Port=2
  Enable : EnablePort
  Subsystem : Subsystem
  Out1 : Outport
  wires:
  vector/1 -> Subsystem/1(vector)
  Subsystem/1(original_vector) -> Out1/1
  vector1/1 -> Subsystem/2(vector1)

== system quadcopter_rotation_subsystem/Mathematical model/Enabled Subsystem1 ==
  time_step : Inport
  Enable : EnablePort
  rotation system : Subsystem
  q : Outport
  wires:
  rotation system/1(q) -> q/1
  time_step/1 -> rotation system/1(time_step)

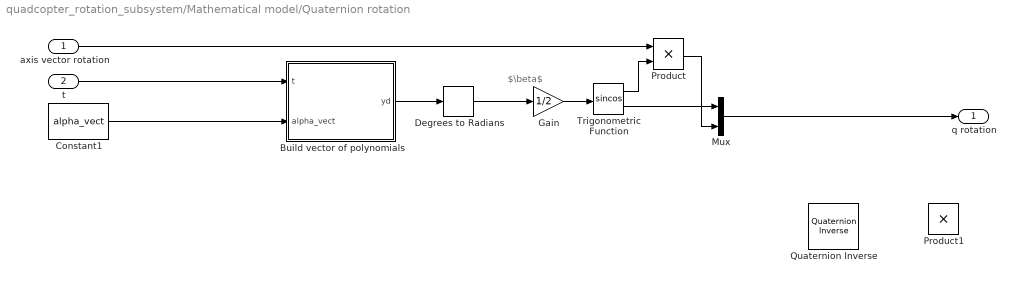
== system quadcopter_rotation_subsystem/Mathematical model/Quaternion rotation  ==
  note: $\beta$
  axis vector rotation : Inport
  t : Inport  Port=2
  Build vector of polynomials : MATLAB Function  TreatAsAtomicUnit=on
  Constant1 : Constant  Value=alpha_vect  VectorParams1D=off
  Degrees to Radians : simulink_extras/Transformations/Degrees to Radians
  Gain : Gain  Gain=1/2
  Mux : Mux  Inputs=2
  Product : Product
  Product1 : Product
  Quaternion Inverse : aerolibutil/Quaternion Inverse
  Trigonometric Function : Trigonometry  Operator=sincos
  q rotation : Outport
  wires:
  Gain/1 -> Trigonometric Function/1
  Trigonometric Function/2 -> Mux/1
  axis vector rotation/1 -> Product/1
  Build vector of polynomials/1(yd) -> Degrees to Radians/1
  Degrees to Radians/1 -> Gain/1
  Trigonometric Function/1 -> Product/2
  Constant1/1 -> Build vector of polynomials/2(alpha_vect)
  Product/1 -> Mux/2
  Mux/1 -> q rotation/1
  t/1 -> Build vector of polynomials/1(t)

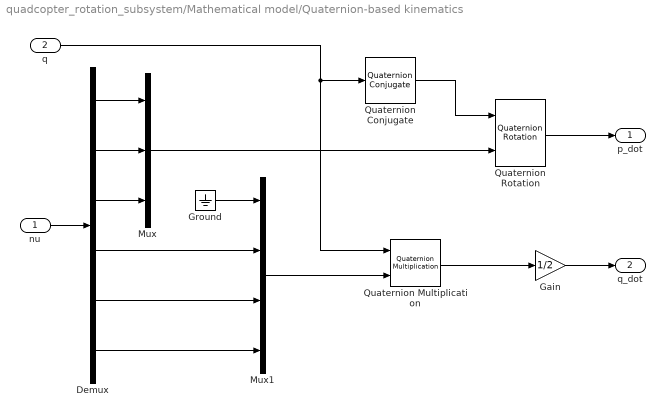
== system quadcopter_rotation_subsystem/Mathematical model/Quaternion-based kinematics ==
  nu : Inport
  q : Inport  Port=2
  Demux : Demux  Outputs=6
  Gain : Gain  Gain=1/2
  Ground : Ground
  Mux : Mux  Inputs=3
  Mux1 : Mux
  Quaternion Conjugate : aerolibutil/Quaternion Conjugate
  Quaternion Multiplication : aerolibutil/Quaternion Multiplication
  Quaternion Rotation : aerolibutil/Quaternion Rotation
  p_dot : Outport
  q_dot : Outport  Port=2
  wires:
  nu/1 -> Demux/1
  Demux/3 -> Mux/3
  Demux/2 -> Mux/2
  Demux/1 -> Mux/1
  Mux/1 -> Quaternion Rotation/2
  Quaternion Rotation/1 -> p_dot/1
  Quaternion Multiplication/1 -> Gain/1
  Gain/1 -> q_dot/1
  Mux1/1 -> Quaternion Multiplication/2
  Demux/4 -> Mux1/2
  Demux/5 -> Mux1/3
  Demux/6 -> Mux1/4
  q/1 -> Quaternion Multiplication/1, Quaternion Conjugate/1
  Ground/1 -> Mux1/1
  Quaternion Conjugate/1 -> Quaternion Rotation/1

== system quadcopter_rotation_subsystem/Mathematical model/Rigid-body dynamics ==
  note: $\nu$
  tau_g : Inport
  tau_p : Inport  Port=2
  Constant : Constant  Value=m
  Constant1 : Constant  Value=Ic  VectorParams1D=off
  Gain : Gain  Gain=inv(Mrb)  Multiplication=Matrix(K*u) (u vector)
  Ground : Ground
  Integrator1 : Integrator  InitialCondition=[0;0;0;0;0;0]
  MATLAB Function : MATLAB Function  TreatAsAtomicUnit=on
  Mux : Mux  Inputs=3
  Sum : Sum  Inputs=|+-+
  nu : Outport
  wires:
  tau_p/1 -> Mux/3
  Constant1/1 -> MATLAB Function/3(Ic)
  Integrator1/1 -> nu/1, MATLAB Function/1(nu)
  Constant/1 -> MATLAB Function/2(m)
  Sum/1 -> Gain/1
  Gain/1 -> Integrator1/1
  Ground/1 -> Mux/2, Mux/1
  Mux/1 -> Sum/1
  MATLAB Function/1(Cnunu) -> Sum/2
  tau_g/1 -> Sum/3

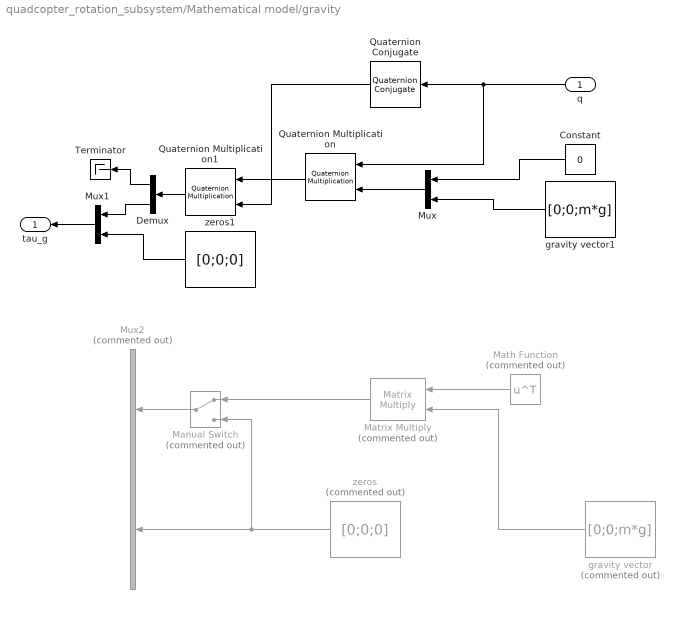
== system quadcopter_rotation_subsystem/Mathematical model/gravity ==
  q : Inport
  Constant : Constant  Value=0
  Demux : Demux  Outputs=[1,3]
  Manual Switch : ManualSwitch  Commented=on
  Math Function : Math  Commented=on  Operator=transpose
  Matrix Multiply : Product  Commented=on  Multiplication=Matrix(*)
  Mux : Mux  Inputs=2
  Mux1 : Mux  Inputs=2
  Mux2 : Mux  Commented=on  Inputs=2
  Quaternion Conjugate : aerolibutil/Quaternion Conjugate
  Quaternion Multiplication : aerolibutil/Quaternion Multiplication
  Quaternion Multiplication1 : aerolibutil/Quaternion Multiplication
  Terminator : Terminator
  gravity vector : Constant  Commented=on  Value=[0;0;m*g]  VectorParams1D=off
  gravity vector1 : Constant  Value=[0;0;m*g]  VectorParams1D=off
  zeros : Constant  Commented=on  Value=[0;0;0]  VectorParams1D=off
  zeros1 : Constant  Value=[0;0;0]  VectorParams1D=off
  tau_g : Outport
  wires:
  Matrix Multiply/1 -> Manual Switch/1
  Manual Switch/1 -> Mux2/1
  gravity vector/1 -> Matrix Multiply/2
  zeros/1 -> Mux2/2, Manual Switch/2
  Math Function/1 -> Matrix Multiply/1
  gravity vector1/1 -> Mux/2
  Constant/1 -> Mux/1
  q/1 -> Quaternion Multiplication/1, Quaternion Conjugate/1
  Mux/1 -> Quaternion Multiplication/2
  Quaternion Multiplication/1 -> Quaternion Multiplication1/1
  Quaternion Conjugate/1 -> Quaternion Multiplication1/2
  zeros1/1 -> Mux1/2
  Mux1/1 -> tau_g/1
  Quaternion Multiplication1/1 -> Demux/1
  Demux/2 -> Mux1/1
  Demux/1 -> Terminator/1

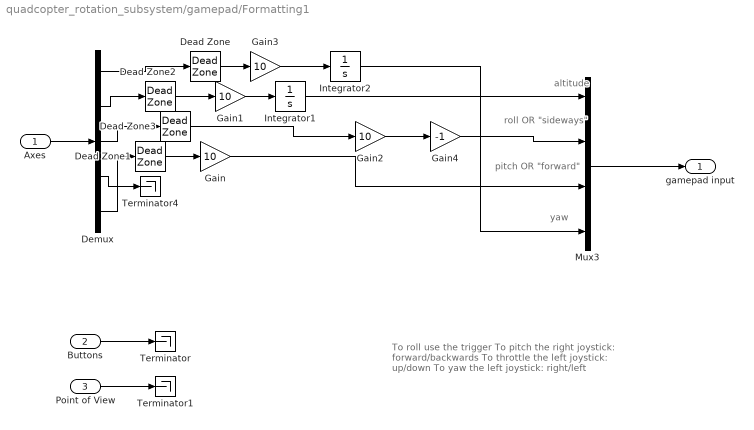
== system quadcopter_rotation_subsystem/gamepad/Formatting1 ==
  note: To roll use the trigger
      | To pitch the right joystick: forward/backwards
      | To throttle the left joystick: up/down
      | To yaw the left joystick: right/left
  note: roll OR "sideways"
  note: altitude
  note: pitch OR "forward"
  note: yaw
  Axes : Inport
  Buttons : Inport  Port=2
  Point of View : Inport  Port=3
  Dead Zone{,1..3} (4 alike) : DeadZone  LowerValue=-0.2  UpperValue=0.2
  Demux : Demux  Outputs=5
  Gain{,1..3} (4 alike) : Gain  Gain=10
  Gain4 : Gain  Gain=-1
  Integrator1 : Integrator  InitialCondition=-17
  Integrator2 : Integrator  InitialCondition=-45
  Mux3 : Mux
  Terminator : Terminator
  Terminator1 : Terminator
  Terminator4 : Terminator
  gamepad input : Outport
  wires:
  Buttons/1 -> Terminator/1
  Axes/1 -> Demux/1
  Demux/3 -> Dead Zone3/1
  Demux/1 -> Dead Zone/1
  Dead Zone1/1 -> Gain/1
  Demux/2 -> Dead Zone2/1
  Dead Zone2/1 -> Gain1/1
  Integrator1/1 -> Mux3/1
  Dead Zone/1 -> Gain3/1
  Integrator2/1 -> Mux3/4
  Dead Zone3/1 -> Gain2/1
  Point of View/1 -> Terminator1/1
  Gain1/1 -> Integrator1/1
  Gain2/1 -> Gain4/1
  Gain/1 -> Mux3/3
  Gain3/1 -> Integrator2/1
  Demux/5 -> Dead Zone1/1
  Demux/4 -> Terminator4/1
  Gain4/1 -> Mux3/2
  Mux3/1 -> gamepad input/1

== system quadcopter_rotation_subsystem/Formatting/Euler to VR/Axis Angle Vector ==
  e0 : Inport
  2 : Gain  Gain=2  SaturateOnIntegerOverflow=on  OutDataTypeStr=Inherit: Same as input  ParamDataTypeStr=Inherit: Same as input
  Constant : Constant  Value=1e-6
  Demux : Demux  Outputs=[1 3 ]
      settings: DisplayOption=none
  Mux : Mux  Inputs=2
  Product : Product  Inputs=*/  InputSameDT=on  SaturateOnIntegerOverflow=on  OutDataTypeStr=Inherit: Same as first input
  Switch : Switch  Criteria=u2 ~= 0  SaturateOnIntegerOverflow=off  InputSameDT=off
  Trigonometric Function : Trigonometry
  Trigonometric Function2 : Trigonometry  Operator=acos
  e0_norm : Outport  VectorParamsAs1DForOutWhenUnconnected=off
  wires:
  Demux/1 -> Trigonometric Function2/1
  Demux/2 -> Product/1
  Mux/1 -> e0_norm/1
  Product/1 -> Mux/1
  2/1 -> Mux/2
  Trigonometric Function/1 -> Switch/1, Switch/2
  Trigonometric Function2/1 -> Trigonometric Function/1, 2/1
  e0/1 -> Demux/1
  Constant/1 -> Switch/3
  Switch/1 -> Product/2

== system quadcopter_rotation_subsystem/Formatting/Euler to VR/Quaternion Normalization ==
  e0 : Inport
  1/2 : Gain  Gain=1/2  SaturateOnIntegerOverflow=on  OutDataTypeStr=Inherit: Same as input  ParamDataTypeStr=Inherit: Same as input
  Demux : Demux  Outputs=[1 3]
      settings: DisplayOption=none
  Mux : Mux  Inputs=2
  Product : Product  InputSameDT=on  SaturateOnIntegerOverflow=on  OutDataTypeStr=Inherit: Same as first input
  Trigonometric Function : Trigonometry
  Trigonometric Function1 : Trigonometry  Operator=cos
  e0_norm : Outport  VectorParamsAs1DForOutWhenUnconnected=off
  wires:
  Trigonometric Function1/1 -> Mux/1
  Demux/2 -> Product/2
  Demux/1 -> 1/2/1
  Mux/1 -> e0_norm/1
  Product/1 -> Mux/2
  Trigonometric Function/1 -> Product/1
  1/2/1 -> Trigonometric Function1/1, Trigonometric Function/1
  e0/1 -> Demux/1

== system quadcopter_rotation_subsystem/Formatting/Euler to VR/Quaternion Normalization1 ==
  e0 : Inport
  1/2 : Gain  Gain=1/2  SaturateOnIntegerOverflow=on  OutDataTypeStr=Inherit: Same as input  ParamDataTypeStr=Inherit: Same as input
  Demux : Demux  Outputs=[1 3]
      settings: DisplayOption=none
  Mux : Mux  Inputs=2
  Product : Product  InputSameDT=on  SaturateOnIntegerOverflow=on  OutDataTypeStr=Inherit: Same as first input
  Trigonometric Function : Trigonometry
  Trigonometric Function1 : Trigonometry  Operator=cos
  e0_norm : Outport  VectorParamsAs1DForOutWhenUnconnected=off
  wires:
  e0/1 -> Demux/1
  1/2/1 -> Trigonometric Function/1, Trigonometric Function1/1
  Trigonometric Function/1 -> Product/1
  Product/1 -> Mux/2
  Mux/1 -> e0_norm/1
  Demux/1 -> 1/2/1
  Demux/2 -> Product/2
  Trigonometric Function1/1 -> Mux/1
